simulink model "parte1Simulink"  (R2021a)
settings: Solver=VariableStepAuto  StartTime=0.0  StopTime=2400  FixedStep=0.1  RelTol=1e-3
values from neighbouring files (symbols this model uses):
  h_e = 0.45    [parte1.m]
  u_e = Q_i/(pi * d^2 * sqrt(2*G*x_e)/4)    [parte1.m]
  x_e = 0.45    [parte1.m]
libraries: cstblocks x4
settings Model: Creator=Cristian  LastModifiedBy=nnobi

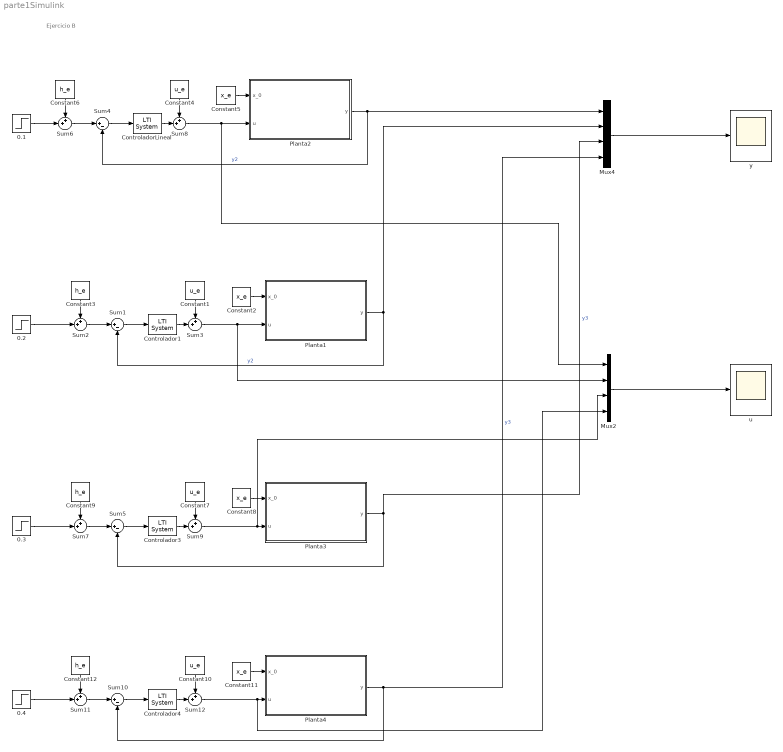
== system parte1Simulink ==
  note: Ejercicio B
  0.1 : Step  Time=60  After=0.1  SampleTime=0
  0.2 : Step  Time=60  After=0.1  SampleTime=0
  0.3 : Step  Time=60  After=0.1
  0.4 : Step  Time=60  After=0.1  SampleTime=0
  Constant{1,4,7,10} (4 alike) : Constant  Value=u_e
  Constant{2,5,8,11} (4 alike) : Constant  Value=x_e
  Constant{3,6,9,12} (4 alike) : Constant  Value=h_e
  Controlador1 : cstblocks/LTI System  sys=cd_fe  IC=[]
  Controlador3 : cstblocks/LTI System  sys=cd_be  IC=[]
  Controlador4 : cstblocks/LTI System  sys=cd_t  IC=[]
  ControladorLineal : cstblocks/LTI System  sys=C  IC=[]
  Mux2 : Mux
  Mux4 : Mux
  Planta1 : Subsystem
  Planta2 : Subsystem
  Planta3 : Subsystem
  Planta4 : Subsystem
  Sum{1,4..5,10} (4 alike) : Sum  Inputs=|+-
  Sum{2..3,6..9,11..12} (8 alike) : Sum  Inputs=++|
  u : Scope
  y : Scope
  wires:
  Constant5/1 -> Planta2/1(x_0)
  Planta2/1(y) -> Sum4/2, Mux4/1  "y2"
  Sum4/1 -> ControladorLineal/1
  Mux2/1 -> u/1
  0.1/1 -> Sum6/2
  Constant6/1 -> Sum6/1
  Sum6/1 -> Sum4/1
  ControladorLineal/1 -> Sum8/2
  Sum8/1 -> Mux2/1, Planta2/2(u)
  Constant4/1 -> Sum8/1
  Mux4/1 -> y/1
  Sum1/1 -> Controlador1/1
  Sum2/1 -> Sum1/1
  Constant3/1 -> Sum2/1
  Constant1/1 -> Sum3/1
  Controlador1/1 -> Sum3/2
  0.2/1 -> Sum2/2
  Planta1/1(y) -> Mux4/2, Sum1/2  "y2"
  Sum3/1 -> Mux2/2, Planta1/2(u)
  Constant2/1 -> Planta1/1(x_0)
  Sum5/1 -> Controlador3/1
  Sum7/1 -> Sum5/1
  Constant9/1 -> Sum7/1
  Constant7/1 -> Sum9/1
  Controlador3/1 -> Sum9/2
  0.3/1 -> Sum7/2
  Planta3/1(y) -> Mux4/3, Sum5/2  "y3"
  Sum9/1 -> Planta3/2(u), Mux2/3
  Constant8/1 -> Planta3/1(x_0)
  Constant11/1 -> Planta4/1(x_0)
  Sum12/1 -> Mux2/4, Planta4/2(u)
  Planta4/1(y) -> Mux4/4, Sum10/2  "y3"
  Constant10/1 -> Sum12/1
  Sum10/1 -> Controlador4/1
  Sum11/1 -> Sum10/1
  Constant12/1 -> Sum11/1
  0.4/1 -> Sum11/2
  Controlador4/1 -> Sum12/2

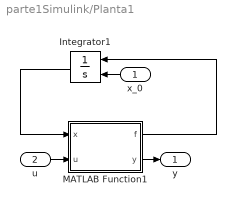
== system parte1Simulink/Planta1 ==
  x_0 : Inport
  u : Inport  Port=2
  Integrator1 : Integrator  InitialConditionSource=external
  MATLAB Function1 : MATLAB Function  TreatAsAtomicUnit=on
  y : Outport
  wires:
  MATLAB Function1/1(f) -> Integrator1/1
  Integrator1/1 -> MATLAB Function1/1(x)
  MATLAB Function1/2(y) -> y/1
  u/1 -> MATLAB Function1/2(u)
  x_0/1 -> Integrator1/2

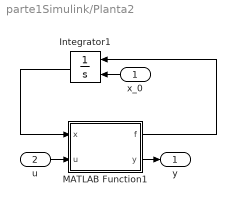
== system parte1Simulink/Planta2 ==
  x_0 : Inport
  u : Inport  Port=2
  Integrator1 : Integrator  InitialConditionSource=external
  MATLAB Function1 : MATLAB Function  TreatAsAtomicUnit=on
  y : Outport
  wires:
  MATLAB Function1/1(f) -> Integrator1/1
  Integrator1/1 -> MATLAB Function1/1(x)
  MATLAB Function1/2(y) -> y/1
  u/1 -> MATLAB Function1/2(u)
  x_0/1 -> Integrator1/2

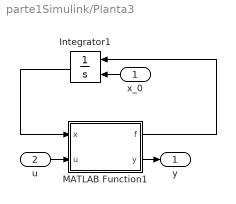
== system parte1Simulink/Planta3 ==
  x_0 : Inport
  u : Inport  Port=2
  Integrator1 : Integrator  InitialConditionSource=external
  MATLAB Function1 : MATLAB Function  TreatAsAtomicUnit=on
  y : Outport
  wires:
  MATLAB Function1/1(f) -> Integrator1/1
  Integrator1/1 -> MATLAB Function1/1(x)
  MATLAB Function1/2(y) -> y/1
  u/1 -> MATLAB Function1/2(u)
  x_0/1 -> Integrator1/2

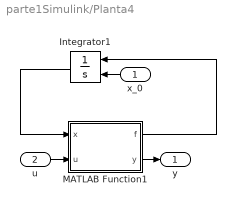
== system parte1Simulink/Planta4 ==
  x_0 : Inport
  u : Inport  Port=2
  Integrator1 : Integrator  InitialConditionSource=external
  MATLAB Function1 : MATLAB Function  TreatAsAtomicUnit=on
  y : Outport
  wires:
  MATLAB Function1/1(f) -> Integrator1/1
  Integrator1/1 -> MATLAB Function1/1(x)
  MATLAB Function1/2(y) -> y/1
  u/1 -> MATLAB Function1/2(u)
  x_0/1 -> Integrator1/2

== matlab function parte1Simulink/Planta3/MATLAB Function1 ==
  data: x input; f output; u input; y output
function [f,y] = fcn(x,u)
G = 9.8;

a_max = 0.4;
h_max = 0.9;
b = 0.1;
d = 0.01065;
Q_i = 8e-3/60;

m = (a_max - b)/h_max;

f = (Q_i - pi * d^2 * sqrt(2*G*x)*u/4 )/(m^2 * x^2 + 2*b*m*x + b^2);

y = x;

== matlab function parte1Simulink/Planta2/MATLAB Function1 ==
  data: x input; f output; u input; y output
function [f,y] = fcn(x,u)
G = 9.8;

a_max = 0.4;
h_max = 0.9;
b = 0.1;
d = 0.01065;
Q_i = 8e-3/60;

m = (a_max - b)/h_max;

f = (Q_i - pi * d^2 * sqrt(2*G*x)*u/4 )/(m^2 * x^2 + 2*b*m*x + b^2);

y = x;

== matlab function parte1Simulink/Planta4/MATLAB Function1 ==
  data: x input; f output; u input; y output
function [f,y] = fcn(x,u)
G = 9.8;

a_max = 0.4;
h_max = 0.9;
b = 0.1;
d = 0.01065;
Q_i = 8e-3/60;

m = (a_max - b)/h_max;

f = (Q_i - pi * d^2 * sqrt(2*G*x)*u/4 )/(m^2 * x^2 + 2*b*m*x + b^2);

y = x;

== matlab function parte1Simulink/Planta1/MATLAB Function1 ==
  data: x input; f output; u input; y output
function [f,y] = fcn(x,u)
G = 9.8;

a_max = 0.4;
h_max = 0.9;
b = 0.1;
d = 0.01065;
Q_i = 8e-3/60;

m = (a_max - b)/h_max;

f = (Q_i - pi * d^2 * sqrt(2*G*x)*u/4 )/(m^2 * x^2 + 2*b*m*x + b^2);

y = x;
